simulink model "adaptiveModelReal"  (R2015a)
settings: Solver=ode3  StartTime=0.0  StopTime=10.0  FixedStep=1/200  RelTol=1e-3
undefined symbols (not defined in the file): Aref, B, Bref, GammaX, P
libraries: PoliArd x6, simulink x4
settings Model: ExtModeTrigDuration=2  Creator=GSavaia  LastModifiedBy=user
settings OptimizationCC: OptimizeModelRefInitCode=on  LifeSpan=1
settings DebuggingCC: UnderspecifiedInitializationDetection=Classic  MergeDetectMultiDrivingBlocksExec=none
settings HardwareCC: ProdLargestAtomicInteger=Long  ProdLargestAtomicFloat=Double  ProdEndianess=LittleEndian  ProdHWDeviceType=ARM Compatible->ARM Cortex
settings RTWCC: SystemTargetFile=realtime.tlc  GenerateMakefile=off  TemplateMakefile=realtime.tmf  Description=Run on Target Hardware  RTWVerbose=off
settings ERTTargetCC: CombineOutputUpdateFcns=off  ExtModeTransport=3  ExtModeMexFile=ext_serial_win32_comm_rtt  ExtModeMexArgs=0 1 9600  ERTSrcFileBannerTemplate=realtime_code_template.cgt  ERTHdrFileBannerTemplate=realtime_code_template.cgt  ERTDataSrcFileTemplate=realtime_code_template.cgt  ERTDataHdrFileTemplate=realtime_code_template.cgt  ERTCustomFileTemplate=realtime_file_process.tlc

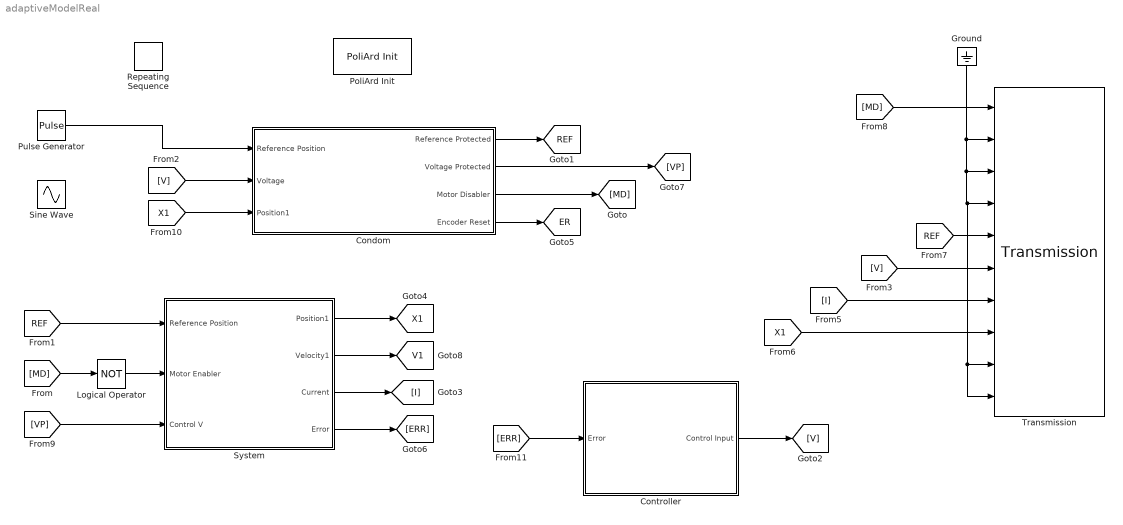
== system adaptiveModelReal ==
  Condom : Subsystem
  Controller : Subsystem
  Ground : Ground
  Logical Operator : Logic  Operator=NOT  AllPortsSameDT=off  OutDataTypeStr=boolean
  PoliArd Init : PoliArd/PoliArd Init
  Pulse Generator : DiscretePulseGenerator  PulseType=Time based  Period=10  PulseWidth=50  PhaseDelay=5
  Repeating Sequence : simulink/Sources/Repeating Sequence  rep_seq_t=[0 5]  rep_seq_y=[0 1]
  Sine Wave : Sin  Amplitude=0  Bias=0.5  Frequency=2*pi  SampleTime=0
  "System " : Subsystem
  Transmission : PoliArd/Transmission  sample_freq=200  sig_to_send=6
  tag scope: ER=global, REF=global, V1=global, X1=global
  wires:
  Logical Operator/1 -> "System "/2(Motor Enabler)
  [MD] -> Logical Operator/1
  Condom/1(Reference Protected) -> [REF]
  [REF] -> "System "/1(Reference Position)
  "System "/3(Current) -> [I]
  [V] -> Condom/2(Voltage)
  [V] -> Transmission/6
  [I] -> Transmission/7
  "System "/1(Position1) -> [X1]
  [REF] -> Transmission/5
  [MD] -> Transmission/1
  [VP] -> "System "/3(Control V)
  [X1] -> Condom/3(Position1)
  [X1] -> Transmission/8
  Controller/1(Control Input) -> [V]
  "System "/4(Error) -> [ERR]
  [ERR] -> Controller/1(Error)
  Condom/2("Voltage Protected ") -> [VP]
  Condom/3(Motor Disabler) -> [MD]
  Condom/4(Encoder Reset) -> [ER]
  Ground/1 -> Transmission/10, Transmission/9, Transmission/4, Transmission/3, Transmission/2
  Pulse Generator/1 -> Condom/1(Reference Position)
  "System "/2(Velocity1) -> [V1]

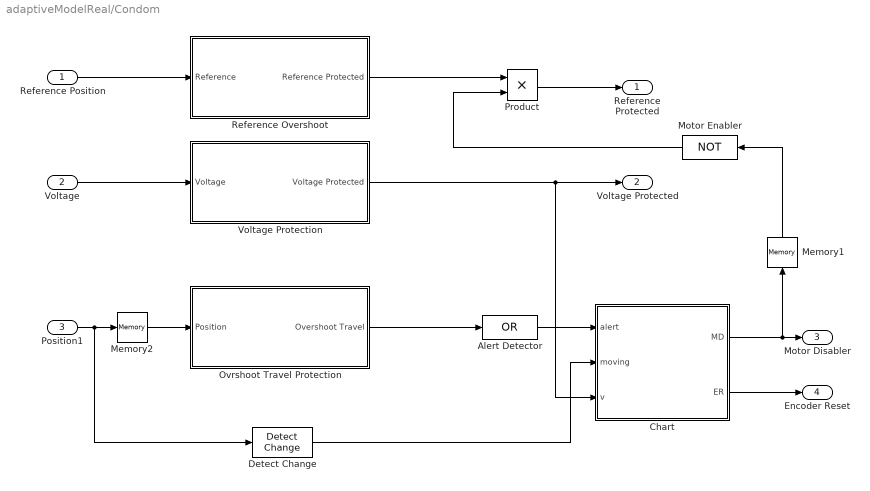
== system adaptiveModelReal/Condom ==
  Reference Position : Inport
  Voltage : Inport  Port=2
  Position1 : Inport  Port=3
  Alert Detector : Logic  Operator=OR  Inputs=1  AllPortsSameDT=off  OutDataTypeStr=boolean
  Chart : Stateflow chart  TreatAsAtomicUnit=on
  Detect Change : simulink/Logic and Bit Operations/Detect Change  vinit=0  InputProcessing=Inherited  OutDataTypeStr=boolean
  Memory1 : Memory
  Memory2 : Memory
  Motor Enabler : Logic  Operator=NOT  Inputs=1  AllPortsSameDT=off  OutDataTypeStr=boolean
  Ovrshoot Travel Protection : Subsystem
  Product : Product
  Reference Overshoot : Subsystem
  Voltage Protection : Subsystem
  Reference Protected : Outport
  "Voltage Protected " : Outport  Port=2
  Motor Disabler : Outport  Port=3
  Encoder Reset : Outport  Port=4
  wires:
  Reference Position/1 -> Reference Overshoot/1("Reference ")
  Memory2/1 -> Ovrshoot Travel Protection/1("Position ")
  Position1/1 -> Detect Change/1, Memory2/1
  Ovrshoot Travel Protection/1(Overshoot Travel) -> Alert Detector/1
  Alert Detector/1 -> Chart/1(alert)
  Detect Change/1 -> Chart/2(moving)
  Chart/1(MD) -> Memory1/1, Motor Disabler/1
  Chart/2(ER) -> Encoder Reset/1
  Voltage/1 -> Voltage Protection/1("Voltage ")
  Voltage Protection/1(Voltage Protected) -> Chart/3(v), "Voltage Protected "/1
  Product/1 -> Reference Protected/1
  Reference Overshoot/1(Reference Protected) -> Product/1
  Motor Enabler/1 -> Product/2
  Memory1/1 -> Motor Enabler/1

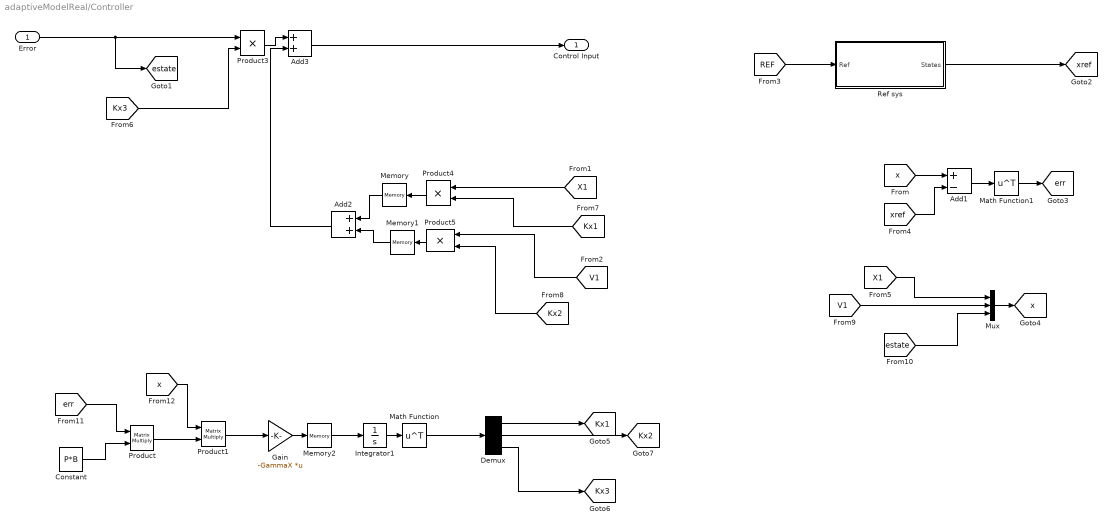
== system adaptiveModelReal/Controller ==
  Error : Inport
  Add1 : Sum  Inputs=+-
  Add2 : Sum
  Add3 : Sum
  Constant : Constant  Value=P*B
  Demux : Demux  Outputs=3
  Gain : Gain  Gain=-GammaX  Multiplication=Matrix(K*u)
  Integrator1 : Integrator
  Math Function : Math  Operator=transpose  SaturateOnIntegerOverflow=on
  Math Function1 : Math  Operator=transpose  SaturateOnIntegerOverflow=on
  Memory : Memory
  Memory1 : Memory
  Memory2 : Memory
  Mux : Mux  Inputs=3
  Product : Product  Multiplication=Matrix(*)
  Product1 : Product  Multiplication=Matrix(*)
  Product3 : Product
  Product4 : Product
  Product5 : Product
  Ref sys : Subsystem
  Control Input : Outport
  tag scope: Kx1=global, Kx2=global, Kx3=global, err=global, estate=global, x=global, xref=global
  wires:
  [Kx3] -> Product3/2
  [Kx1] -> Product4/2
  [Kx2] -> Product5/2
  Error/1 -> [estate], Product3/1
  Product3/1 -> Add3/1
  Add2/1 -> Add3/2
  Add3/1 -> Control Input/1
  [X1] -> Product4/1
  [V1] -> Product5/1
  Ref sys/1(States) -> [xref]
  [REF] -> Ref sys/1(Ref)
  [x] -> Add1/1
  [xref] -> Add1/2
  Add1/1 -> Math Function1/1
  Math Function1/1 -> [err]
  [X1] -> Mux/1
  [V1] -> Mux/2
  [estate] -> Mux/3
  Mux/1 -> [x]
  [err] -> Product/1
  Constant/1 -> Product/2
  Product/1 -> Product1/2
  [x] -> Product1/1
  Product1/1 -> Gain/1
  Integrator1/1 -> Math Function/1
  Math Function/1 -> Demux/1
  Demux/1 -> [Kx1]
  Demux/3 -> [Kx3]
  Demux/2 -> [Kx2]
  Product4/1 -> Memory/1
  Memory/1 -> Add2/1
  Product5/1 -> Memory1/1
  Memory1/1 -> Add2/2
  Gain/1 -> Memory2/1
  Memory2/1 -> Integrator1/1

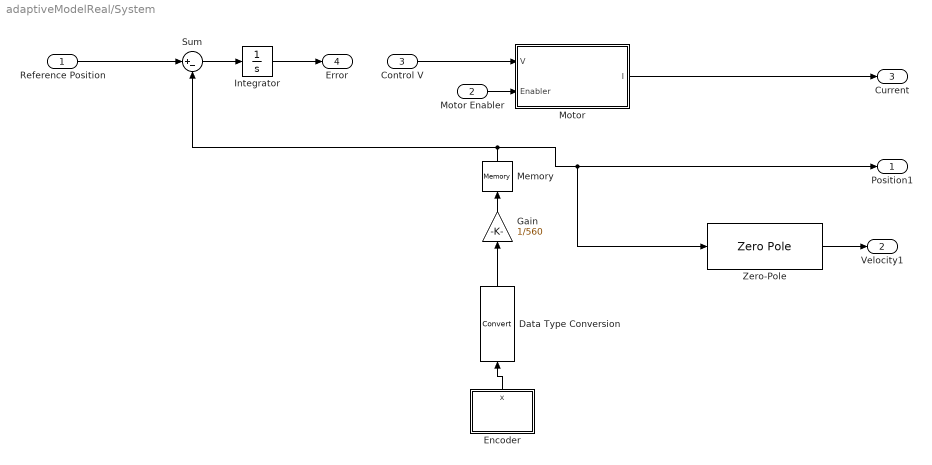
== system adaptiveModelReal/System  ==
  Reference Position : Inport
  Motor Enabler : Inport  Port=2
  Control V : Inport  Port=3
  Data Type Conversion : DataTypeConversion
  "Encoder " : Subsystem
  Gain : Gain  Gain=1/560
  Integrator : Integrator
  Memory : Memory
  Motor : Subsystem
  Sum : Sum  Inputs=|+-
  Zero-Pole : ZeroPole  Zeros=[0]  Poles=[-100,-150]  Gain=100*150
  Position1 : Outport
  Velocity1 : Outport  Port=2
  Current : Outport  Port=3
  Error : Outport  Port=4
  wires:
  Reference Position/1 -> Sum/1
  Motor/1(I) -> Current/1
  Motor Enabler/1 -> Motor/2(Enabler)
  Control V/1 -> Motor/1(V)
  Sum/1 -> Integrator/1
  Integrator/1 -> Error/1
  Zero-Pole/1 -> Velocity1/1
  Data Type Conversion/1 -> Gain/1
  "Encoder "/1(x) -> Data Type Conversion/1
  Gain/1 -> Memory/1
  Memory/1 -> Zero-Pole/1, Position1/1, Sum/2

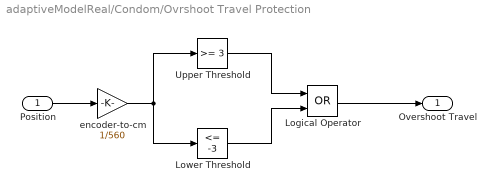
== system adaptiveModelReal/Condom/Ovrshoot Travel Protection ==
  "Position " : Inport
  Logical Operator : Logic  Operator=OR  AllPortsSameDT=off  OutDataTypeStr=boolean
  Lower Threshold : simulink/Logic and Bit Operations/Compare To Constant  relop=<=  const=-3  OutDataTypeStr=boolean
  Upper Threshold : simulink/Logic and Bit Operations/Compare To Constant  relop=>=  const=3  OutDataTypeStr=boolean
  encoder-to-cm : Gain  Gain=1/560
  Overshoot Travel : Outport
  wires:
  Logical Operator/1 -> Overshoot Travel/1
  Lower Threshold/1 -> Logical Operator/2
  Upper Threshold/1 -> Logical Operator/1
  "Position "/1 -> encoder-to-cm/1
  encoder-to-cm/1 -> Lower Threshold/1, Upper Threshold/1

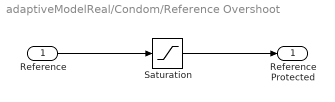
== system adaptiveModelReal/Condom/Reference Overshoot ==
  "Reference " : Inport
  Saturation : Saturate  UpperLimit=3  LowerLimit=-3
  Reference Protected : Outport
  wires:
  Saturation/1 -> Reference Protected/1
  "Reference "/1 -> Saturation/1

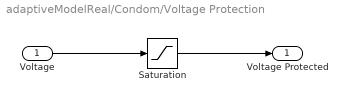
== system adaptiveModelReal/Condom/Voltage Protection ==
  "Voltage " : Inport
  Saturation : Saturate  UpperLimit=5  LowerLimit=-5
  Voltage Protected : Outport
  wires:
  Saturation/1 -> Voltage Protected/1
  "Voltage "/1 -> Saturation/1

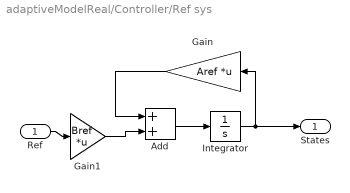
== system adaptiveModelReal/Controller/Ref sys ==
  Ref : Inport
  Add : Sum
  Gain : Gain  Gain=Aref  Multiplication=Matrix(K*u)
  Gain1 : Gain  Gain=Bref  Multiplication=Matrix(K*u)
  Integrator : Integrator
  States : Outport
  wires:
  Gain/1 -> Add/1
  Gain1/1 -> Add/2
  Add/1 -> Integrator/1
  Ref/1 -> Gain1/1
  Integrator/1 -> States/1, Gain/1

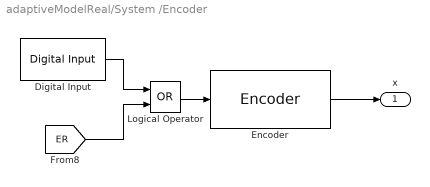
== system adaptiveModelReal/System /Encoder  ==
  Digital Input : PoliArd/Digital Input  DI_pin=2  DIsample=1/200
  Encoder : PoliArd/Encoder  EncoderID=1  dt_enc=1/200
  Logical Operator : Logic  Operator=OR  AllPortsSameDT=off  OutDataTypeStr=boolean
  x : Outport
  wires:
  Encoder/1 -> x/1
  Digital Input/1 -> Logical Operator/1
  [ER] -> Logical Operator/2
  Logical Operator/1 -> Encoder/1

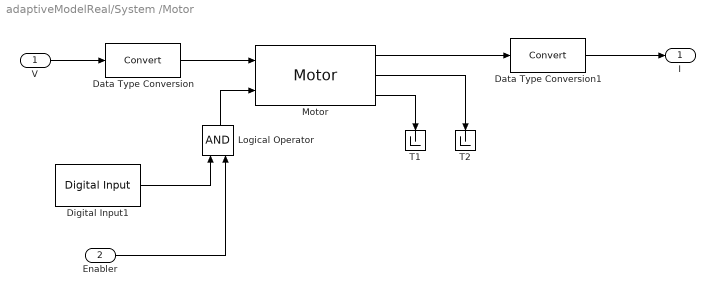
== system adaptiveModelReal/System /Motor ==
  V : Inport
  Enabler : Inport  Port=2
  Data Type Conversion : DataTypeConversion
  Data Type Conversion1 : DataTypeConversion
  Digital Input1 : PoliArd/Digital Input  DI_pin=3  DIsample=1/200
  Logical Operator : Logic  AllPortsSameDT=off  OutDataTypeStr=boolean
  Motor : PoliArd/Motor  MotorID=2  DC_bus_mask=12  dt_mot=1/200
  T1 : Terminator
  T2 : Terminator
  I : Outport
  wires:
  Data Type Conversion/1 -> Motor/1
  V/1 -> Data Type Conversion/1
  Motor/3 -> T1/1
  Motor/2 -> T2/1
  Motor/1 -> Data Type Conversion1/1
  Data Type Conversion1/1 -> I/1
  Enabler/1 -> Logical Operator/2
  Logical Operator/1 -> Motor/2
  Digital Input1/1 -> Logical Operator/1

== stateflow chart adaptiveModelReal/Condom/Chart ==
  state OK
    entry:
    MD=0;
    ER=0;
  state ALERT
    entry:
    MD=1;
  state RESTORE
    entry:
    MD=1;
    ER=1
  (default) -> OK
  OK -> ALERT : [alert==1]
  RESTORE -> OK : [v==0]
  ALERT -> RESTORE : [moving==0]
  data: MD output; ER output; alert input; moving input; v input
